simulink model "automata_learning"  (R2022a)
settings: Solver=FixedStepAuto  StartTime=0.0  StopTime=10.0  FixedStep=0.05  RelTol=1e-3
settings Model: Creator=diego  LastModifiedBy=diego

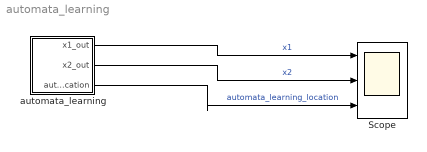
== system automata_learning ==
  Scope : Scope  NumInputPorts=3
  automata_learning : Stateflow chart  TreatAsAtomicUnit=on
  wires:
  automata_learning/1(x1_out) -> Scope/1  "x1"
  automata_learning/2(x2_out) -> Scope/2  "x2"
  automata_learning/3(automata_learning_location) -> Scope/3  "automata_learning_location"

== stateflow chart automata_learning/automata_learning ==
  settings: updateMethod=CONTINUOUS
  state loc1
    du:
    x1_dot = 0.00000000000001887379141862766 * x1 - 0.0000000000000009829601348143184 * x2 + 1.0;
    x2_dot = x1 - 0.0000000000000011102230246251565 * x2 - 0.000000000000013968860790303239;
    x1_out=x1;
    x2_out=x2;
    automata_learning_location =1;
  state loc2
    du:
    x1_dot = 0.0000000000000004198234099811604 - 0.049999999999954525 * x2 - 0.000000000000013322676295501878 * x1;
    x2_dot = 0.00000000000005091228954312111 * x1 + 0.00000000000005773159728050814 * x2 + 1.0;
    x1_out=x1;
    x2_out=x2;
    automata_learning_location =2;
  loc1 -> loc2 : [0.0000005511 * x2 - 0.2482 * x1 + 1.0 < 0.0]
  (default) -> loc1 : {x1 = 0.0;
      | x2 = 0.0;}
  loc2 -> loc1 : [43.09132960916031 * x1 + 0.021145646542095164 * x2 + 1.0 < 0.0 && -75.02048562094569 * x1 - 0.1991395009226835 * x2 + 1.0 > 0.0]
  data: x1_out output; x1 local; x2_out output; x2 local; automata_learning_location output
  data x1 settings: updateMethod=SF_CONTINUOUS_TIME_DATA
  data x2 settings: updateMethod=SF_CONTINUOUS_TIME_DATA
